simulink subsystem "IdealOPAmp"  (R2019b)
settings: Solver=VariableStepAuto  StartTime=0.0  StopTime=10.0  RelTol=1e-3
settings Model: Creator=ykamatan  LastModifiedBy=ykamatan
settings DebuggingCC: UnconnectedInputMsg=none  UnconnectedOutputMsg=none  UnconnectedLineMsg=none  SFMachineParentedDataDiag=error
settings ModelReferenceCC: EnableRefExpFcnMdlSchedulingChecks=off
settings RTWCC: Description=Generic Real-Time Target

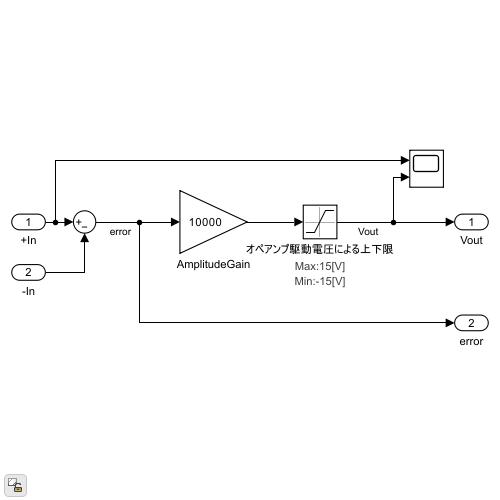
[thumbnail: Simulink's stored preview of the top-level diagram]
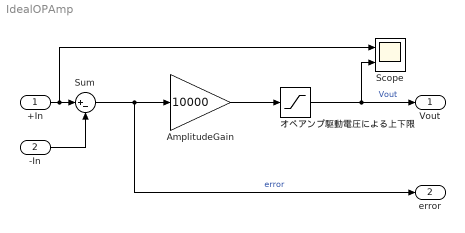
== system IdealOPAmp ==
  +In : Inport
  -In : Inport  Port=2
  AmplitudeGain : Gain  Gain=10000
  Scope : Scope  NumInputPorts=2
  Sum : Sum  Inputs=|+-
  オペアンプ駆動電圧による上下限 : Saturate  UpperLimit=15  LowerLimit=-15
      settings: AttributesFormatString=|
      | Max:%<UpperLimit>[V]
      | Min:%<LowerLimit>[V]
  Vout : Outport
  error : Outport  Port=2
  wires:
  AmplitudeGain/1 -> オペアンプ駆動電圧による上下限/1
  オペアンプ駆動電圧による上下限/1 -> Vout/1, Scope/2  "Vout"
  +In/1 -> Sum/1, Scope/1
  Sum/1 -> AmplitudeGain/1, error/1  "error"
  -In/1 -> Sum/2
